simulink model "SIM_nonlinear_LQR"  (R2023a)
settings: Solver=ode23t  StartTime=0.0  StopTime=20  MaxStep=1e-4  RelTol=1e-3
values from neighbouring files (symbols this model uses):
  Kr = sqrt(Q(1, 1)/R)    [param.m]
undefined symbols (not defined in the file or in its folder): K
settings Model: Creator=edzel  LastModifiedBy=edzel

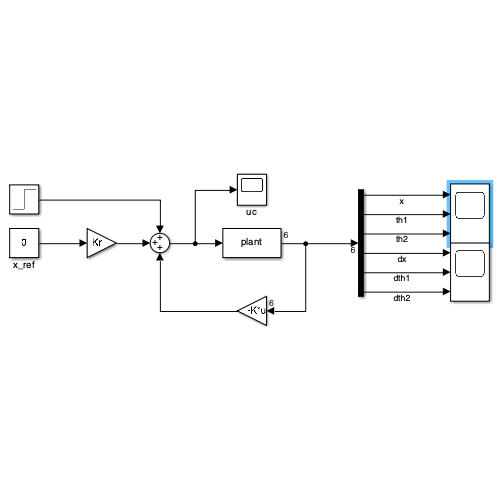
[thumbnail: Simulink's stored preview of the top-level diagram]
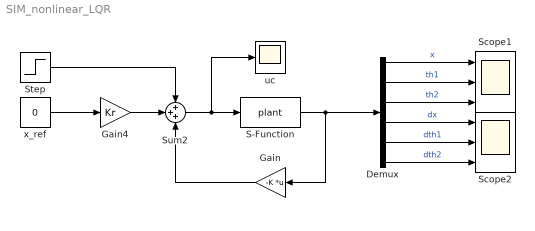
== system SIM_nonlinear_LQR ==
  Demux : Demux  Outputs=6
  Gain : Gain  Gain=-K  Multiplication=Matrix(K*u)
  Gain4 : Gain  Gain=Kr
  S-Function : S-Function  FunctionName=plant  Parameters=CoeF1, CoeF2, CoeF3, theta1_rad, theta2_rad  SFunctionDeploymentMode=off  EnableBusSupport=off
  Scope1 : Scope  NumInputPorts=3
  Scope2 : Scope  NumInputPorts=3
  Step : Step  Time=10  After=0.5  SampleTime=0
  Sum2 : Sum  Inputs=+++
  uc : Scope
  x_ref : Constant  Value=0
  wires:
  Demux/5 -> Scope2/2  "dth1"
  Demux/3 -> Scope1/3  "th2"
  Demux/1 -> Scope1/1  "x"
  Demux/2 -> Scope1/2  "th1"
  Demux/4 -> Scope2/1  "dx"
  Demux/6 -> Scope2/3  "dth2"
  S-Function/1 -> Demux/1, Gain/1
  Sum2/1 -> uc/1, S-Function/1
  x_ref/1 -> Gain4/1
  Step/1 -> Sum2/1
  Gain4/1 -> Sum2/2
  Gain/1 -> Sum2/3
